simulink model "main_PETC"  (R2021a)
settings: Solver=VariableStepAuto  StartTime=0.0  StopTime=10  FixedStep=1e-4  RelTol=1e-3
InitFcn:
  | run('Parameter.m')
values from neighbouring files (symbols this model uses):
  cp = 1    [Parameter.m]
  cv = 5    [Parameter.m]
  cw = 5    [Parameter.m]
  fref = 60    [Parameter.m]
  Lc1 = 0.35e-3    (= 0.00035)    [Parameter.m]
  Lc2 = 0.35e-3    (= 0.00035)    [Parameter.m]
  Lc3 = 0.35e-3    (= 0.00035)    [Parameter.m]
  Lc4 = 0.35e-3    (= 0.00035)    [Parameter.m]
  Lt12 = 318e-6    (= 0.000318)    [Parameter.m]
  Lt23 = 1847e-6    (= 0.001847)    [Parameter.m]
  Lt34 = 318e-6    (= 0.000318)    [Parameter.m]
  Mp1 = 9.4e-5    (= 9.4e-05)    [Parameter.m]
  Mp2 = 9.4e-5    (= 9.4e-05)    [Parameter.m]
  Mp3 = 12.5e-5    (= 0.000125)    [Parameter.m]
  Mp4 = 12.5e-5    (= 0.000125)    [Parameter.m]
  Nq1 = 1.3e-3    (= 0.0013)    [Parameter.m]
  Nq2 = 1.3e-3    (= 0.0013)    [Parameter.m]
  Nq3 = 1.5e-3    (= 0.0015)    [Parameter.m]
  Nq4 = 1.5e-3    (= 0.0015)    [Parameter.m]
  Rc1 = 0.03    [Parameter.m]
  Rc2 = 0.03    [Parameter.m]
  Rc3 = 0.03    [Parameter.m]
  Rc4 = 0.03    [Parameter.m]
  Rt12 = 0.23    [Parameter.m]
  Rt23 = 0.35    [Parameter.m]
  Rt34 = 0.23    [Parameter.m]
  t2 = 1    [Parameter.m]    (also in wvpq_PETC.m)
  t3 = 10    [Parameter.m]
  t4 = 20    [Parameter.m]    (also in wvpq_PETC.m = 21)
  t5 = 35    [Parameter.m]    (also in wvpq_PETC.m = 33)
  t6 = 40    [Parameter.m]    (also in wvpq_PETC.m = 35)
  Uo = 220*sqrt(2)    [Parameter.m]
  vref = 380    [Parameter.m]
  wc = 31.4    [Parameter.m]
  wref = 2*pi*fref    (= 376.991118431)    [Parameter.m]
undefined symbols (not defined in the file or in its folder): gcbh, sps_rtmsupport
libraries: spsControlledVoltageSourceLib x12, spsAlphaBetaZerotodq0Lib x12, eeGeneralControl x8, spsThreePhaseSeriesRLCBranchLib x7, spsGroundLib x4, spsThreePhaseVIMeasurementLib x4, spsThreePhaseBreakerLib x4, spsPLL3phLib x4, spsThreePhaseSeriesRLCLoadLib x3, spspowerguiLib x1
(part 1 of 2)
settings Model: Creator=Li Ding  LastModifiedBy=服务器

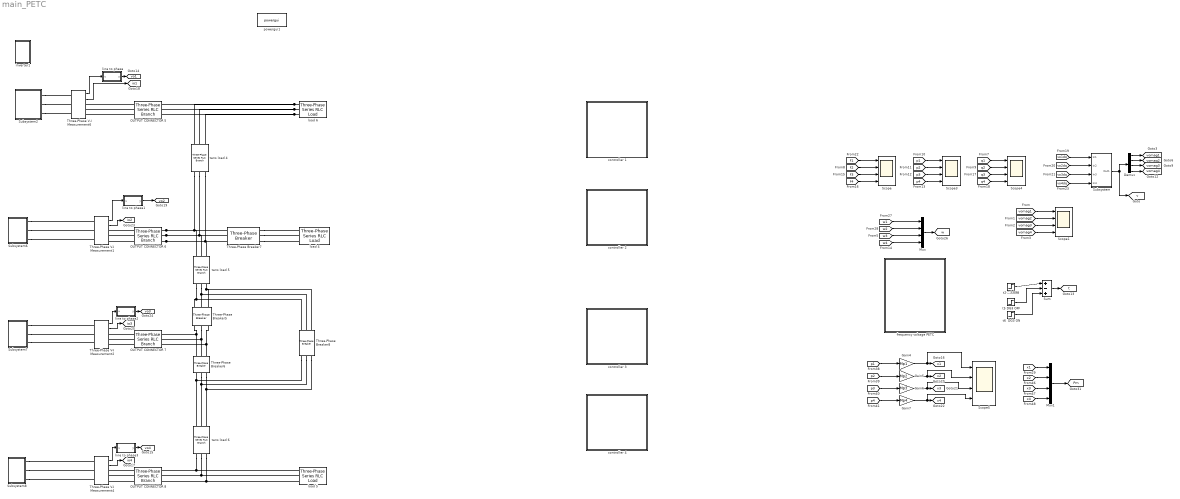
== system main_PETC ==
  Demux : Demux
  Gain4 : Gain  Gain=Mp1
  Gain5 : Gain  Gain=Mp2
  Gain6 : Gain  Gain=Mp3
  Gain7 : Gain  Gain=Mp4
  Mux : Mux
  Mux1 : Mux
  OUTPUT CONNECTOR 5 : spsThreePhaseSeriesRLCBranchLib/Three-Phase Series RLC Branch  LConnTagsString=A|B|C  RConnTagsString=A|B|C  BranchType=RL  Resistance=Rc1  Inductance=Lc1  Capacitance=1e-6  Measurements=None
  OUTPUT CONNECTOR 6 : spsThreePhaseSeriesRLCBranchLib/Three-Phase Series RLC Branch  LConnTagsString=A|B|C  RConnTagsString=A|B|C  BranchType=RL  Resistance=Rc2  Inductance=Lc2  Capacitance=1e-6  Measurements=None
  OUTPUT CONNECTOR 7 : spsThreePhaseSeriesRLCBranchLib/Three-Phase Series RLC Branch  LConnTagsString=A|B|C  RConnTagsString=A|B|C  BranchType=RL  Resistance=Rc3  Inductance=Lc3  Capacitance=1e-6  Measurements=None
  OUTPUT CONNECTOR 8 : spsThreePhaseSeriesRLCBranchLib/Three-Phase Series RLC Branch  LConnTagsString=A|B|C  RConnTagsString=A|B|C  BranchType=RL  Resistance=Rc4  Inductance=Lc4  Capacitance=1e-6  Measurements=None
  Scope{,1,3..5} (5 alike) : Scope  NumInputPorts=4
  Subsystem : Subsystem
  Subsystem2 : Subsystem
  Subsystem6 : Subsystem
  Subsystem7 : Subsystem
  Subsystem8 : Subsystem
  Sum : Sum  Inputs=|+-+
  Three-Phase V-I Measurement{1..2,4,6} (4 alike) : spsThreePhaseVIMeasurementLib/Three-Phase V-I Measurement  VoltageMeasurement=phase-to-phase  SetLabelV=off  LabelV=Vabc  Vpu=off  VpuLL=off  CurrentMeasurement=yes  SetLabelI=off  LabelI=Iabc  Ipu=off  Pbase=100e6  Vbase=500e3  OutputType=Complex  PhasorSimulation=off  PSBequivalent=0
  Three-Phase Breaker5 : spsThreePhaseBreakerLib/Three-Phase Breaker  InitialState=closed  SwitchA=on  SwitchB=on  SwitchC=on  SwitchTimes=[t5 t6]  External=off  BreakerResistance=0.01  SnubberResistance=1e6  SnubberCapacitance=inf  Measurements=None
  Three-Phase Breaker6 : spsThreePhaseBreakerLib/Three-Phase Breaker  InitialState=closed  SwitchA=on  SwitchB=on  SwitchC=on  SwitchTimes=[t5 t6]  External=off  BreakerResistance=0.01  SnubberResistance=1e6  SnubberCapacitance=inf  Measurements=None
  Three-Phase Breaker7 : spsThreePhaseBreakerLib/Three-Phase Breaker  InitialState=open  SwitchA=on  SwitchB=on  SwitchC=on  SwitchTimes=[t3 t4]  External=off  BreakerResistance=0.01  SnubberResistance=1e6  SnubberCapacitance=inf  Measurements=None
  Three-Phase Breaker8 : spsThreePhaseBreakerLib/Three-Phase Breaker  InitialState=open  SwitchA=on  SwitchB=on  SwitchC=on  SwitchTimes=[t5 t6]  External=off  BreakerResistance=0.01  SnubberResistance=1e6  SnubberCapacitance=inf  Measurements=None
  controller 1 : Subsystem
  controller 2 : Subsystem
  controller 3 : Subsystem
  controller 4 : Subsystem
  frequency voltage PETC : Subsystem
  inverter1 : Subsystem
  line to phase : MATLAB Function  TreatAsAtomicUnit=on
  line to phase1 : MATLAB Function  TreatAsAtomicUnit=on
  line to phase2 : MATLAB Function  TreatAsAtomicUnit=on
  line to phase3 : MATLAB Function  TreatAsAtomicUnit=on
  load 4 : spsThreePhaseSeriesRLCLoadLib/Three-Phase Series RLC Load  LConnTagsString=A|B|C  Configuration=Y (grounded)  NominalVoltage=vref  Vabc=[1e3 1e3 1e3]  Vabcp=[1e3 1e3 1e3]  NominalFrequency=fref  UnbalancedPower=off  ActivePower=PL2  InductivePower=QL2  CapacitivePower=0  Pabc=[10e3 9e3 11e3]  QLabc=[100 90 110]  QCabc=[100 90 110]  Pabcp=[10e3 9e3 11e3]  QLabcp=[100 90 110]  QCabcp=[100 90 110]  Measurements=None  LoadType=constant Z
  load 5 : spsThreePhaseSeriesRLCLoadLib/Three-Phase Series RLC Load  LConnTagsString=A|B|C  Configuration=Y (grounded)  NominalVoltage=vref  Vabc=[1e3 1e3 1e3]  Vabcp=[1e3 1e3 1e3]  NominalFrequency=fref  UnbalancedPower=off  ActivePower=PL4  InductivePower=QL4  CapacitivePower=0  Pabc=[10e3 9e3 11e3]  QLabc=[100 90 110]  QCabc=[100 90 110]  Pabcp=[10e3 9e3 11e3]  QLabcp=[100 90 110]  QCabcp=[100 90 110]  Measurements=None  LoadType=constant Z
  load 6 : spsThreePhaseSeriesRLCLoadLib/Three-Phase Series RLC Load  LConnTagsString=A|B|C  Configuration=Y (grounded)  NominalVoltage=vref  Vabc=[1e3 1e3 1e3]  Vabcp=[1e3 1e3 1e3]  NominalFrequency=fref  UnbalancedPower=off  ActivePower=PL1  InductivePower=QL1  CapacitivePower=0  Pabc=[10e3 9e3 11e3]  QLabc=[100 90 110]  QCabc=[100 90 110]  Pabcp=[10e3 9e3 11e3]  QLabcp=[100 90 110]  QCabcp=[100 90 110]  Measurements=None  LoadType=constant Z
  powergui1 : spspowerguiLib/powergui  Priority=1  SimulationMode=Discrete  SampleTime=50e-6  frequency=60  Iterations=50  frequencyindice=0  Pbase=100e6  ErrMax=1e-4  UnitsV=kV  UnitsW=MW  buscounter=0  FunctionMessages=off  echomessages=off  EnableUseOfTLC=off  CurrentSourceSwitches=off  DisableSnubberDevices=off  DisableRonSwitches=off  DisableVfSwitches=off  DisplayEquations=off  AutomaticDiscreteSolvers=off  SolverType=Tustin/Backward Euler (TBE)  Interpol=off  ExternalGateDelay=off  methode=off  Ts=100  x0status=blocks  SPID=on  SwTol=0  HookPort=off  NonlinearTolerance=1e-4  nMaxIteration=100  ContinueOnMaxIteration=off  RestoreLinks=warning  ResistiveCurrentMeasurement=off  Frange=[0:2:500]  Ylog=off  Xlog=on  ShowGrid=off  save=off  variable=ZData  structure=0  ZoomFFT=off  StartTime=0.0  cycles=1  DisplayStyle=1  fundamental=60  FreqAxis=off  MaxFrequency=1000  frequencyindicesteady=1  RmsSteady=1  display=off
  t2-二次控制 : Step  Time=t2  SampleTime=0
  t5 DG3 OFF : Step  Time=t5  SampleTime=0
  t6  DG3 ON : Step  Time=t6  SampleTime=0
  tans load 4 : spsThreePhaseSeriesRLCBranchLib/Three-Phase Series RLC Branch  LConnTagsString=A|B|C  RConnTagsString=A|B|C  BranchType=RL  Resistance=Rt12  Inductance=Lt12  Capacitance=1e-6  Measurements=None
  tans load 5 : spsThreePhaseSeriesRLCBranchLib/Three-Phase Series RLC Branch  LConnTagsString=A|B|C  RConnTagsString=A|B|C  BranchType=RL  Resistance=Rt23  Inductance=Lt23  Capacitance=1e-6  Measurements=None
  tans load 6 : spsThreePhaseSeriesRLCBranchLib/Three-Phase Series RLC Branch  LConnTagsString=A|B|C  RConnTagsString=A|B|C  BranchType=RL  Resistance=Rt34  Inductance=Lt34  Capacitance=1e-6  Measurements=None
  tag scope: Pm=global, io1=global, io2=global, io3=global, io4=global, t=global, v=global, vo1=global, vo2=global, vo3=global, vo4=global, vomag1=global, vomag2=global, vomag3=global, vomag4=global, w=global, x1=global, x2=global, x3=global, x4=global
  wires:
  [f3] -> Scope/3
  [f2] -> Scope/2
  [f1] -> Scope/1
  [f4] -> Scope/4
  [p4] -> Scope3/4
  [q1] -> Scope4/1
  [q4] -> Scope4/4
  [p2] -> Scope3/2
  [q2] -> Scope4/2
  [p1] -> Scope3/1
  [p3] -> Scope3/3
  [q3] -> Scope4/3
  [w1] -> Mux/1
  [w2] -> Mux/2
  [w3] -> Mux/3
  [w4] -> Mux/4
  Mux/1 -> [w]
  [p1] -> Gain4/1
  [p2] -> Gain5/1
  [p3] -> Gain6/1
  [p4] -> Gain7/1
  Gain7/1 -> Scope5/4, [x4]
  Gain6/1 -> Scope5/3, [x3]
  Gain5/1 -> Scope5/2, [x2]
  Gain4/1 -> Scope5/1, [x1]
  [x4] -> Mux1/4
  [x1] -> Mux1/1
  Mux1/1 -> [Pm]
  [x2] -> Mux1/2
  [x3] -> Mux1/3
  Demux/4 -> [vomag4]
  [vo3dq] -> Subsystem/3(In3)
  Demux/2 -> [vomag2]
  [vo1dq] -> Subsystem/1(In1)
  Subsystem/1(Out1) -> [v], Demux/1
  [vo2dq] -> Subsystem/2(In2)
  Demux/1 -> [vomag1]
  [vo4dq] -> Subsystem/4(In4)
  Demux/3 -> [vomag3]
  [vomag4] -> Scope1/4
  [vomag3] -> Scope1/3
  [vomag2] -> Scope1/2
  [vomag1] -> Scope1/1
  Sum/1 -> [t]
  t2-二次控制/1 -> Sum/1
  t5 DG3 OFF/1 -> Sum/2
  t6  DG3 ON/1 -> Sum/3
  Three-Phase V-I Measurement6/2 -> [io1]
  Three-Phase V-I Measurement4/1 -> line to phase3/1(u)
  Three-Phase V-I Measurement1/2 -> [io2]
  Three-Phase V-I Measurement6/1 -> line to phase/1(u)
  line to phase1/1(y) -> [vo2]
  Three-Phase V-I Measurement4/2 -> [io4]
  Three-Phase V-I Measurement1/1 -> line to phase1/1(u)
  line to phase/1(y) -> [vo1]
  line to phase2/1(y) -> [vo3]
  Three-Phase V-I Measurement2/1 -> line to phase2/1(u)
  line to phase3/1(y) -> [vo4]
  Three-Phase V-I Measurement2/2 -> [io3]
  connections:
  OUTPUT CONNECTOR 6/RConn2 -- tans load 4/RConn2 -- tans load 5/LConn2 -- Three-Phase Breaker7/LConn2
  OUTPUT CONNECTOR 6/RConn3 -- tans load 4/RConn3 -- tans load 5/LConn3 -- Three-Phase Breaker7/LConn3
  OUTPUT CONNECTOR 6/RConn1 -- tans load 4/RConn1 -- tans load 5/LConn1 -- Three-Phase Breaker7/LConn1
  tans load 5/RConn1 -- Three-Phase Breaker8/LConn1 -- Three-Phase Breaker5/LConn1
  load 5/LConn1 -- tans load 6/RConn1 -- OUTPUT CONNECTOR 8/RConn1
  load 5/LConn3 -- tans load 6/RConn3 -- OUTPUT CONNECTOR 8/RConn3
  load 5/LConn2 -- tans load 6/RConn2 -- OUTPUT CONNECTOR 8/RConn2
  Three-Phase Breaker5/RConn3 -- OUTPUT CONNECTOR 7/RConn3 -- Three-Phase Breaker6/LConn3
  load 6/LConn3 -- OUTPUT CONNECTOR 5/RConn3 -- tans load 4/LConn3
  load 6/LConn1 -- OUTPUT CONNECTOR 5/RConn1 -- tans load 4/LConn1
  tans load 5/RConn2 -- Three-Phase Breaker8/LConn2 -- Three-Phase Breaker5/LConn2
  tans load 5/RConn3 -- Three-Phase Breaker8/LConn3 -- Three-Phase Breaker5/LConn3
  Three-Phase Breaker6/LConn2 -- OUTPUT CONNECTOR 7/RConn2 -- Three-Phase Breaker5/RConn2
  load 6/LConn2 -- OUTPUT CONNECTOR 5/RConn2 -- tans load 4/LConn2
  Three-Phase Breaker5/RConn1 -- OUTPUT CONNECTOR 7/RConn1 -- Three-Phase Breaker6/LConn1
  Subsystem2/LConn2 -- Three-Phase V-I Measurement6/LConn2
  OUTPUT CONNECTOR 8/LConn1 -- Three-Phase V-I Measurement4/RConn1
  Subsystem2/LConn1 -- Three-Phase V-I Measurement6/LConn1
  Three-Phase Breaker6/RConn3 -- Three-Phase Breaker8/RConn3 -- tans load 6/LConn3
  Subsystem8/LConn1 -- Three-Phase V-I Measurement4/LConn1
  OUTPUT CONNECTOR 8/LConn3 -- Three-Phase V-I Measurement4/RConn3
  OUTPUT CONNECTOR 6/LConn3 -- Three-Phase V-I Measurement1/RConn3
  Subsystem7/LConn1 -- Three-Phase V-I Measurement2/LConn1
  Three-Phase Breaker7/RConn2 -- load 4/LConn2
  Subsystem6/LConn1 -- Three-Phase V-I Measurement1/LConn1
  Subsystem7/LConn3 -- Three-Phase V-I Measurement2/LConn3
  Subsystem6/LConn2 -- Three-Phase V-I Measurement1/LConn2
  Three-Phase Breaker7/RConn1 -- load 4/LConn1
  OUTPUT CONNECTOR 7/LConn3 -- Three-Phase V-I Measurement2/RConn3
  OUTPUT CONNECTOR 7/LConn1 -- Three-Phase V-I Measurement2/RConn1
  Three-Phase Breaker7/RConn3 -- load 4/LConn3
  Subsystem6/LConn3 -- Three-Phase V-I Measurement1/LConn3
  Three-Phase Breaker6/RConn2 -- Three-Phase Breaker8/RConn2 -- tans load 6/LConn2
  Subsystem8/LConn3 -- Three-Phase V-I Measurement4/LConn3
  OUTPUT CONNECTOR 5/LConn2 -- Three-Phase V-I Measurement6/RConn2
  OUTPUT CONNECTOR 8/LConn2 -- Three-Phase V-I Measurement4/RConn2
  OUTPUT CONNECTOR 7/LConn2 -- Three-Phase V-I Measurement2/RConn2
  Subsystem7/LConn2 -- Three-Phase V-I Measurement2/LConn2
  Subsystem2/LConn3 -- Three-Phase V-I Measurement6/LConn3
  OUTPUT CONNECTOR 6/LConn1 -- Three-Phase V-I Measurement1/RConn1
  OUTPUT CONNECTOR 5/LConn3 -- Three-Phase V-I Measurement6/RConn3
  OUTPUT CONNECTOR 5/LConn1 -- Three-Phase V-I Measurement6/RConn1
  Subsystem8/LConn2 -- Three-Phase V-I Measurement4/LConn2
  OUTPUT CONNECTOR 6/LConn2 -- Three-Phase V-I Measurement1/RConn2
  tans load 6/LConn1 -- Three-Phase Breaker8/RConn1 -- Three-Phase Breaker6/RConn1

== system main_PETC/Subsystem ==
  In1 : Inport
  In2 : Inport  Port=2
  In3 : Inport  Port=3
  In4 : Inport  Port=4
  Mux : Mux
  Scope : Scope
  Selector{,1..3} (4 alike) : Selector  InputPortWidth=2  IndexOptions=Index vector (dialog)  Indices=[1]  OutputSizes=1
  Transfer Fcn{,2,4,6} (4 alike) : TransferFcn  Numerator=[200]  Denominator=[1 200]
  Out1 : Outport
  wires:
  Selector1/1 -> Transfer Fcn2/1
  Selector3/1 -> Transfer Fcn6/1
  In4/1 -> Selector3/1
  Selector2/1 -> Transfer Fcn4/1
  Mux/1 -> Out1/1
  In3/1 -> Selector2/1
  In2/1 -> Selector1/1
  In1/1 -> Selector/1
  Transfer Fcn/1 -> Mux/1
  Transfer Fcn2/1 -> Mux/2
  Transfer Fcn4/1 -> Mux/3
  Transfer Fcn6/1 -> Mux/4
  Selector/1 -> Scope/1, Transfer Fcn/1

== system main_PETC/Subsystem2 ==
  Controlled Voltage Source : spsControlledVoltageSourceLib/Controlled Voltage Source  Initialize=on  Source_Type=AC  Amplitude=Uo  Phase=0  Frequency=fref  Measurements=None
  Controlled Voltage Source1 : spsControlledVoltageSourceLib/Controlled Voltage Source  Initialize=on  Source_Type=AC  Amplitude=Uo  Phase=120  Frequency=fref  Measurements=None
  Controlled Voltage Source2 : spsControlledVoltageSourceLib/Controlled Voltage Source  Initialize=on  Source_Type=AC  Amplitude=Uo  Phase=240  Frequency=fref  Measurements=None
  Demux : Demux  Outputs=3
  Ground : spsGroundLib/Ground  LConnTagsString=a
  +1 : PMIOPort  Side=Left
  +2 : PMIOPort  Port=2  Side=Left
  +3 : PMIOPort  Port=3  Side=Left
  wires:
  Demux/1 -> Controlled Voltage Source/1
  Demux/2 -> Controlled Voltage Source1/1
  Demux/3 -> Controlled Voltage Source2/1
  [VOL1] -> Demux/1
  connections:
  Controlled Voltage Source/RConn1 -- +1/RConn1
  Controlled Voltage Source1/RConn1 -- +2/RConn1
  Controlled Voltage Source2/RConn1 -- +3/RConn1
  Controlled Voltage Source2/LConn1 -- Ground/LConn1 -- Controlled Voltage Source/LConn1 -- Controlled Voltage Source1/LConn1

== system main_PETC/Subsystem6 ==
  Controlled Voltage Source : spsControlledVoltageSourceLib/Controlled Voltage Source  Initialize=on  Source_Type=AC  Amplitude=Uo  Phase=0  Frequency=fref  Measurements=None
  Controlled Voltage Source1 : spsControlledVoltageSourceLib/Controlled Voltage Source  Initialize=on  Source_Type=AC  Amplitude=Uo  Phase=120  Frequency=fref  Measurements=None
  Controlled Voltage Source2 : spsControlledVoltageSourceLib/Controlled Voltage Source  Initialize=on  Source_Type=AC  Amplitude=Uo  Phase=240  Frequency=fref  Measurements=None
  Demux : Demux  Outputs=3
  Ground : spsGroundLib/Ground  LConnTagsString=a
  +1 : PMIOPort  Side=Left
  +2 : PMIOPort  Port=2  Side=Left
  +3 : PMIOPort  Port=3  Side=Left
  wires:
  Demux/1 -> Controlled Voltage Source/1
  Demux/2 -> Controlled Voltage Source1/1
  Demux/3 -> Controlled Voltage Source2/1
  [VOL2] -> Demux/1
  connections:
  Controlled Voltage Source/RConn1 -- +1/RConn1
  Controlled Voltage Source1/RConn1 -- +2/RConn1
  Controlled Voltage Source2/RConn1 -- +3/RConn1
  Controlled Voltage Source/LConn1 -- Controlled Voltage Source1/LConn1 -- Controlled Voltage Source2/LConn1 -- Ground/LConn1

== system main_PETC/Subsystem7 ==
  Controlled Voltage Source : spsControlledVoltageSourceLib/Controlled Voltage Source  Initialize=on  Source_Type=AC  Amplitude=Uo  Phase=0  Frequency=fref  Measurements=None
  Controlled Voltage Source1 : spsControlledVoltageSourceLib/Controlled Voltage Source  Initialize=on  Source_Type=AC  Amplitude=Uo  Phase=120  Frequency=fref  Measurements=None
  Controlled Voltage Source2 : spsControlledVoltageSourceLib/Controlled Voltage Source  Initialize=on  Source_Type=AC  Amplitude=Uo  Phase=240  Frequency=fref  Measurements=None
  Demux : Demux  Outputs=3
  Ground : spsGroundLib/Ground  LConnTagsString=a
  +1 : PMIOPort  Side=Left
  +2 : PMIOPort  Port=2  Side=Left
  +3 : PMIOPort  Port=3  Side=Left
  wires:
  Demux/1 -> Controlled Voltage Source/1
  Demux/2 -> Controlled Voltage Source1/1
  Demux/3 -> Controlled Voltage Source2/1
  [VOL3] -> Demux/1
  connections:
  Controlled Voltage Source/RConn1 -- +1/RConn1
  Controlled Voltage Source1/RConn1 -- +2/RConn1
  Controlled Voltage Source2/RConn1 -- +3/RConn1
  Controlled Voltage Source/LConn1 -- Controlled Voltage Source1/LConn1 -- Controlled Voltage Source2/LConn1 -- Ground/LConn1

== system main_PETC/Subsystem8 ==
  Controlled Voltage Source : spsControlledVoltageSourceLib/Controlled Voltage Source  Initialize=on  Source_Type=AC  Amplitude=Uo  Phase=0  Frequency=fref  Measurements=None
  Controlled Voltage Source1 : spsControlledVoltageSourceLib/Controlled Voltage Source  Initialize=on  Source_Type=AC  Amplitude=Uo  Phase=120  Frequency=fref  Measurements=None
  Controlled Voltage Source2 : spsControlledVoltageSourceLib/Controlled Voltage Source  Initialize=on  Source_Type=AC  Amplitude=Uo  Phase=240  Frequency=fref  Measurements=None
  Demux : Demux  Outputs=3
  Ground : spsGroundLib/Ground  LConnTagsString=a
  +1 : PMIOPort  Side=Left
  +2 : PMIOPort  Port=2  Side=Left
  +3 : PMIOPort  Port=3  Side=Left
  wires:
  Demux/1 -> Controlled Voltage Source/1
  Demux/2 -> Controlled Voltage Source1/1
  Demux/3 -> Controlled Voltage Source2/1
  [VOL4] -> Demux/1
  connections:
  Controlled Voltage Source/RConn1 -- +1/RConn1
  Controlled Voltage Source1/RConn1 -- +2/RConn1
  Controlled Voltage Source2/RConn1 -- +3/RConn1
  Controlled Voltage Source/LConn1 -- Controlled Voltage Source1/LConn1 -- Controlled Voltage Source2/LConn1 -- Ground/LConn1

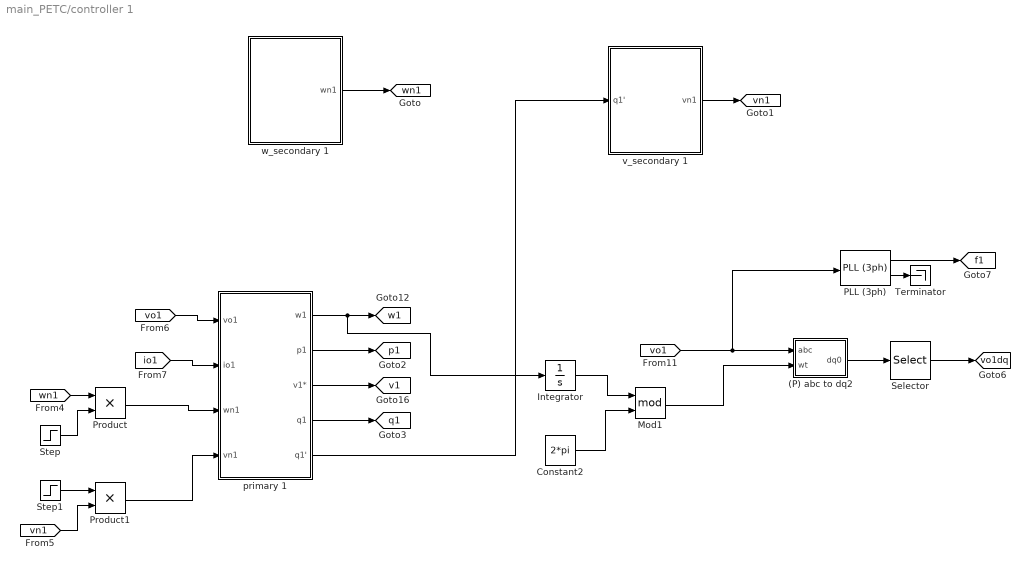
== system main_PETC/controller 1 ==
  (P) abc to dq2 : Subsystem  AncestorBlock=powerlib_meascontrol/Transformations/abc to dq0  DialogController=POWERSYS.PowerSysDialog  LoadFcn=sps_rtmsupport('LoadFcn', gcbh);  StartFcn=sps_rtmsupport('StartFcn', gcbh);  StopFcn=sps_rtmsupport('StopFcn', gcbh);  mask(abc to dq0 Transformation){Alignment=90 degrees behind phase A axis}
      mask prompts: Alignment "Rotating frame alignment at wt=0:"
      mask help:
      | Perform a Park transformation from a three-phase (abc) signal to a dq0 rotating reference frame. Angular position of the rotating frame is given by input wt (rad).
      |
      | When the rotating frame alignment at wt=0 is 90 degrees behind phase A axis, a positive-sequence signal with Mag=1 & Phase=0 degrees yields the following dq values: d=1, q=0.
      mask init:
      | str=cat(2,gcb,'/Alpha-Beta-Zero to dq0');
      | if Alignment==1
      |     set_param(str,'Alignment','Aligned with phase A axis');
      | else
      |     set_param(str,'Alignment','90 degrees behind phase A axis');
      | end
      settings: CopyFcn=sps_rtmsupport('CopyFcn', gcbh);  DeleteFcn=sps_rtmsupport('DeleteFcn', gcbh);  UndoDeleteFcn=sps_rtmsupport('UndoDeleteFcn', gcbh);  ModelCloseFcn=sps_rtmsupport('ModelCloseFcn', gcbh);  PreSaveFcn=sps_rtmsupport('PreSaveFcn', gcbh);  PostSaveFcn=sps_rtmsupport('PostSaveFcn', gcbh);  NameChangeFcn=sps_rtmsupport('NameChangeFcn', gcbh);  PreCopyFcn=sps_rtmsupport('PreCopyFcn', gcbh);  OpenFcn=sps_rtmsupport('OpenFcn', gcbh, [1]);  CloseFcn=sps_rtmsupport('CloseFcn', gcbh);  PreDeleteFcn=sps_rtmsupport('PreDeleteFcn', gcbh);
      mask Help: helpview(psbhelp);
      mask TypeOptions Alignment: Aligned with phase A axis | 90 degrees behind phase A axis
      mask Display:
      | plot([0 1], [0,1])
      | port_label('input', 1, 'abc')
      | port_label('input', 2, 'wt')
      | port_label('output', 1, 'dq0')
  Constant2 : Constant  Value=2*pi
  Integrator : Integrator
  Mod1 : Math  Operator=mod  SaturateOnIntegerOverflow=on
  PLL (3ph) : spsPLL3phLib/PLL (3ph)  Fmin=45  Par_Init=[0, fref]  ParK=[180, 3200, 1]  TcD=1e-4  MaxRateChangeFreq=12  FilterCutOffFreq=25  Ts=0  AGC=on
  Product : Product
  Product1 : Product
  Selector : Selector  InputPortWidth=3  IndexOptions=Index vector (dialog)  Indices=[1 2]  OutputSizes=1
  Step : Step  Time=t2  SampleTime=0
  Step1 : Step  Time=t2  SampleTime=0
  Terminator : Terminator
  primary 1 : Subsystem
  v_secondary 1 : Subsystem
  w_secondary 1 : Subsystem
  tag scope: f1=global, p1=global, q1=global, v1=global, vn1=global, vo1dq=global, w1=global, wn1=global
  wires:
  w_secondary 1/1(wn1) -> [wn1]
  v_secondary 1/1(vn1) -> [vn1]
  primary 1/5(q1') -> v_secondary 1/1(q1')
  PLL (3ph)/2 -> Terminator/1
  Product/1 -> primary 1/3(wn1)
  (P) abc to dq2/1(dq0) -> Selector/1
  primary 1/3(v1*) -> [v1]
  Mod1/1 -> (P) abc to dq2/2(wt)
  Step/1 -> Product/2
  primary 1/4(q1) -> [q1]
  [vn1] -> Product1/2
  Product1/1 -> primary 1/4(vn1)
  primary 1/1(w1) -> Integrator/1, [w1]
  [vo1] -> (P) abc to dq2/1(abc), PLL (3ph)/1
  Constant2/1 -> Mod1/2
  Step1/1 -> Product1/1
  Integrator/1 -> Mod1/1
  [vo1] -> primary 1/1(vo1)
  primary 1/2(p1) -> [p1]
  PLL (3ph)/1 -> [f1]
  Selector/1 -> [vo1dq]
  [wn1] -> Product/1
  [io1] -> primary 1/2(io1)

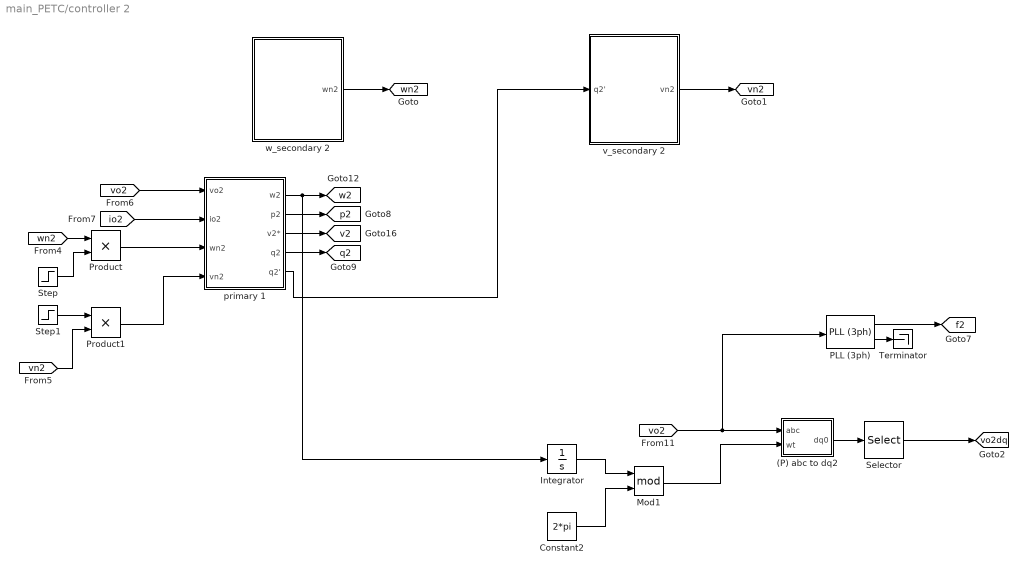
== system main_PETC/controller 2 ==
  (P) abc to dq2 : Subsystem  AncestorBlock=powerlib_meascontrol/Transformations/abc to dq0  DialogController=POWERSYS.PowerSysDialog  LoadFcn=sps_rtmsupport('LoadFcn', gcbh);  StartFcn=sps_rtmsupport('StartFcn', gcbh);  StopFcn=sps_rtmsupport('StopFcn', gcbh);  mask(abc to dq0 Transformation){Alignment=90 degrees behind phase A axis}
      mask prompts: Alignment "Rotating frame alignment at wt=0:"
      mask help:
      | Perform a Park transformation from a three-phase (abc) signal to a dq0 rotating reference frame. Angular position of the rotating frame is given by input wt (rad).
      |
      | When the rotating frame alignment at wt=0 is 90 degrees behind phase A axis, a positive-sequence signal with Mag=1 & Phase=0 degrees yields the following dq values: d=1, q=0.
      mask init:
      | str=cat(2,gcb,'/Alpha-Beta-Zero to dq0');
      | if Alignment==1
      |     set_param(str,'Alignment','Aligned with phase A axis');
      | else
      |     set_param(str,'Alignment','90 degrees behind phase A axis');
      | end
      settings: CopyFcn=sps_rtmsupport('CopyFcn', gcbh);  DeleteFcn=sps_rtmsupport('DeleteFcn', gcbh);  UndoDeleteFcn=sps_rtmsupport('UndoDeleteFcn', gcbh);  ModelCloseFcn=sps_rtmsupport('ModelCloseFcn', gcbh);  PreSaveFcn=sps_rtmsupport('PreSaveFcn', gcbh);  PostSaveFcn=sps_rtmsupport('PostSaveFcn', gcbh);  NameChangeFcn=sps_rtmsupport('NameChangeFcn', gcbh);  PreCopyFcn=sps_rtmsupport('PreCopyFcn', gcbh);  OpenFcn=sps_rtmsupport('OpenFcn', gcbh, [1]);  CloseFcn=sps_rtmsupport('CloseFcn', gcbh);  PreDeleteFcn=sps_rtmsupport('PreDeleteFcn', gcbh);
      mask Help: helpview(psbhelp);
      mask TypeOptions Alignment: Aligned with phase A axis | 90 degrees behind phase A axis
      mask Display:
      | plot([0 1], [0,1])
      | port_label('input', 1, 'abc')
      | port_label('input', 2, 'wt')
      | port_label('output', 1, 'dq0')
  Constant2 : Constant  Value=2*pi
  Integrator : Integrator
  Mod1 : Math  Operator=mod  SaturateOnIntegerOverflow=on
  PLL (3ph) : spsPLL3phLib/PLL (3ph)  Fmin=45  Par_Init=[0, 60]  ParK=[180, 3200, 1]  TcD=1e-4  MaxRateChangeFreq=12  FilterCutOffFreq=25  Ts=0  AGC=on
  Product : Product
  Product1 : Product
  Selector : Selector  InputPortWidth=3  IndexOptions=Index vector (dialog)  Indices=[1 2]  OutputSizes=1
  Step : Step  Time=t2  SampleTime=0
  Step1 : Step  Time=t2  SampleTime=0
  Terminator : Terminator
  primary 1 : Subsystem
  v_secondary 2 : Subsystem
  w_secondary 2 : Subsystem
  tag scope: f2=global, p2=global, q2=global, v2=global, vn2=global, vo2dq=global, w2=global, wn2=global
  wires:
  w_secondary 2/1(wn2) -> [wn2]
  v_secondary 2/1(vn2) -> [vn2]
  PLL (3ph)/2 -> Terminator/1
  primary 1/3(v2*) -> [v2]
  Step1/1 -> Product1/1
  Step/1 -> Product/2
  primary 1/2(p2) -> [p2]
  Product1/1 -> primary 1/4(vn2)
  [vn2] -> Product1/2
  primary 1/4(q2) -> [q2]
  [vo2] -> primary 1/1(vo2)
  PLL (3ph)/1 -> [f2]
  [io2] -> primary 1/2(io2)
  Product/1 -> primary 1/3(wn2)
  primary 1/5(q2') -> v_secondary 2/1(q2')
  Integrator/1 -> Mod1/1
  [wn2] -> Product/1
  (P) abc to dq2/1(dq0) -> Selector/1
  Constant2/1 -> Mod1/2
  Mod1/1 -> (P) abc to dq2/2(wt)
  [vo2] -> (P) abc to dq2/1(abc), PLL (3ph)/1
  primary 1/1(w2) -> [w2], Integrator/1
  Selector/1 -> [vo2dq]

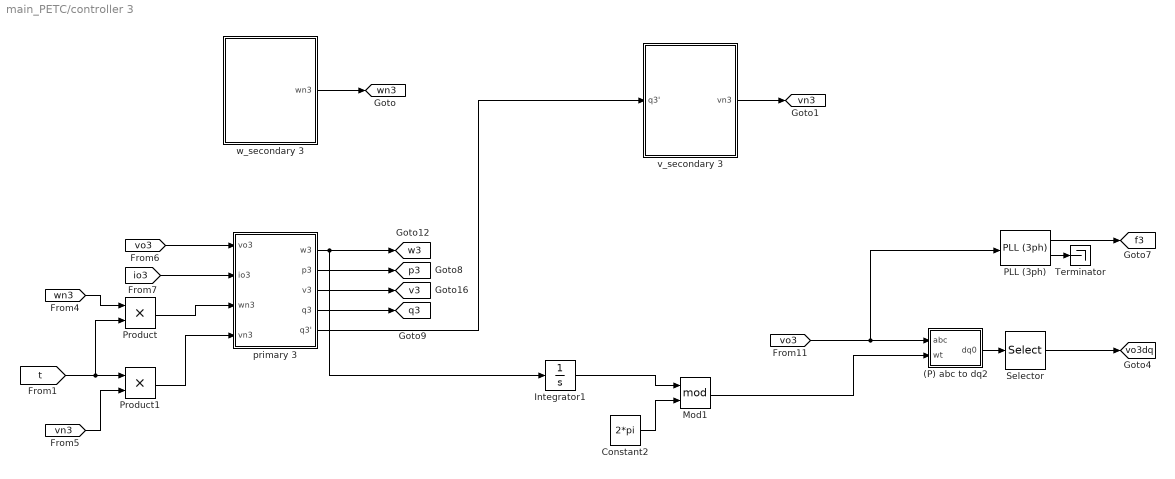
== system main_PETC/controller 3 ==
  (P) abc to dq2 : Subsystem  AncestorBlock=powerlib_meascontrol/Transformations/abc to dq0  DialogController=POWERSYS.PowerSysDialog  LoadFcn=sps_rtmsupport('LoadFcn', gcbh);  StartFcn=sps_rtmsupport('StartFcn', gcbh);  StopFcn=sps_rtmsupport('StopFcn', gcbh);  mask(abc to dq0 Transformation){Alignment=90 degrees behind phase A axis}
      mask prompts: Alignment "Rotating frame alignment at wt=0:"
      mask help:
      | Perform a Park transformation from a three-phase (abc) signal to a dq0 rotating reference frame. Angular position of the rotating frame is given by input wt (rad).
      |
      | When the rotating frame alignment at wt=0 is 90 degrees behind phase A axis, a positive-sequence signal with Mag=1 & Phase=0 degrees yields the following dq values: d=1, q=0.
      mask init:
      | str=cat(2,gcb,'/Alpha-Beta-Zero to dq0');
      | if Alignment==1
      |     set_param(str,'Alignment','Aligned with phase A axis');
      | else
      |     set_param(str,'Alignment','90 degrees behind phase A axis');
      | end
      settings: CopyFcn=sps_rtmsupport('CopyFcn', gcbh);  DeleteFcn=sps_rtmsupport('DeleteFcn', gcbh);  UndoDeleteFcn=sps_rtmsupport('UndoDeleteFcn', gcbh);  ModelCloseFcn=sps_rtmsupport('ModelCloseFcn', gcbh);  PreSaveFcn=sps_rtmsupport('PreSaveFcn', gcbh);  PostSaveFcn=sps_rtmsupport('PostSaveFcn', gcbh);  NameChangeFcn=sps_rtmsupport('NameChangeFcn', gcbh);  PreCopyFcn=sps_rtmsupport('PreCopyFcn', gcbh);  OpenFcn=sps_rtmsupport('OpenFcn', gcbh, [1]);  CloseFcn=sps_rtmsupport('CloseFcn', gcbh);  PreDeleteFcn=sps_rtmsupport('PreDeleteFcn', gcbh);
      mask Help: helpview(psbhelp);
      mask TypeOptions Alignment: Aligned with phase A axis | 90 degrees behind phase A axis
      mask Display:
      | plot([0 1], [0,1])
      | port_label('input', 1, 'abc')
      | port_label('input', 2, 'wt')
      | port_label('output', 1, 'dq0')
  Constant2 : Constant  Value=2*pi
  Integrator1 : Integrator
  Mod1 : Math  Operator=mod  SaturateOnIntegerOverflow=on
  PLL (3ph) : spsPLL3phLib/PLL (3ph)  Fmin=45  Par_Init=[0, 60]  ParK=[180, 3200, 1]  TcD=1e-4  MaxRateChangeFreq=12  FilterCutOffFreq=25  Ts=0  AGC=on
  Product : Product
  Product1 : Product
  Selector : Selector  InputPortWidth=3  IndexOptions=Index vector (dialog)  Indices=[1 2]  OutputSizes=1
  Terminator : Terminator
  primary 3 : Subsystem
  v_secondary 3 : Subsystem
  w_secondary 3 : Subsystem
  tag scope: f3=global, p3=global, q3=global, v3=global, vn3=global, vo3dq=global, w3=global, wn3=global
  wires:
  w_secondary 3/1(wn3) -> [wn3]
  v_secondary 3/1(vn3) -> [vn3]
  Integrator1/1 -> Mod1/1
  primary 3/5(q3') -> v_secondary 3/1(q3')
  [vo3] -> (P) abc to dq2/1(abc), PLL (3ph)/1
  [t] -> Product/2, Product1/1
  Mod1/1 -> (P) abc to dq2/2(wt)
  Constant2/1 -> Mod1/2
  primary 3/4(q3) -> [q3]
  Selector/1 -> [vo3dq]
  primary 3/3(v3) -> [v3]
  (P) abc to dq2/1(dq0) -> Selector/1
  PLL (3ph)/1 -> [f3]
  [vo3] -> primary 3/1(vo3)
  PLL (3ph)/2 -> Terminator/1
  primary 3/2(p3) -> [p3]
  Product/1 -> primary 3/3(wn3)
  primary 3/1(w3) -> [w3], Integrator1/1
  Product1/1 -> primary 3/4(vn3)
  [wn3] -> Product/1
  [vn3] -> Product1/2
  [io3] -> primary 3/2(io3)

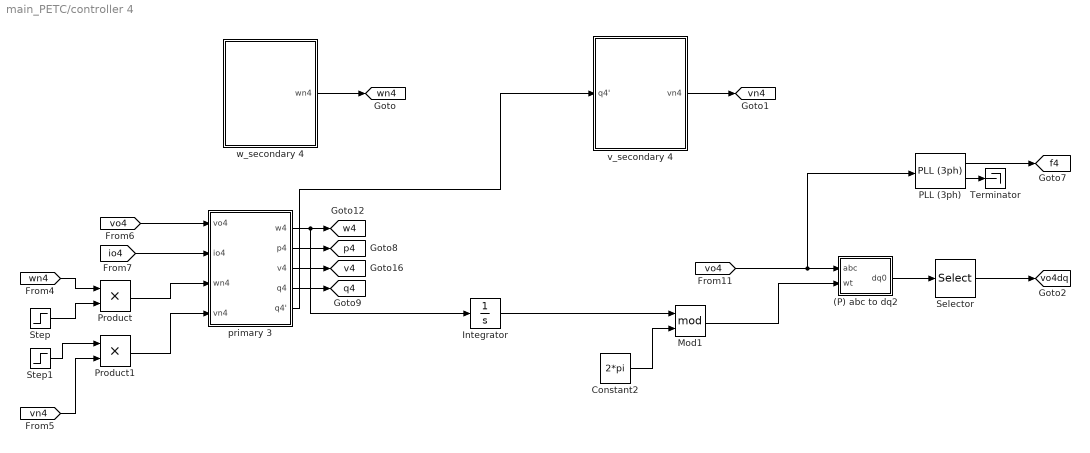
== system main_PETC/controller 4 ==
  (P) abc to dq2 : Subsystem  AncestorBlock=powerlib_meascontrol/Transformations/abc to dq0  DialogController=POWERSYS.PowerSysDialog  LoadFcn=sps_rtmsupport('LoadFcn', gcbh);  StartFcn=sps_rtmsupport('StartFcn', gcbh);  StopFcn=sps_rtmsupport('StopFcn', gcbh);  mask(abc to dq0 Transformation){Alignment=90 degrees behind phase A axis}
      mask prompts: Alignment "Rotating frame alignment at wt=0:"
      mask help:
      | Perform a Park transformation from a three-phase (abc) signal to a dq0 rotating reference frame. Angular position of the rotating frame is given by input wt (rad).
      |
      | When the rotating frame alignment at wt=0 is 90 degrees behind phase A axis, a positive-sequence signal with Mag=1 & Phase=0 degrees yields the following dq values: d=1, q=0.
      mask init:
      | str=cat(2,gcb,'/Alpha-Beta-Zero to dq0');
      | if Alignment==1
      |     set_param(str,'Alignment','Aligned with phase A axis');
      | else
      |     set_param(str,'Alignment','90 degrees behind phase A axis');
      | end
      settings: CopyFcn=sps_rtmsupport('CopyFcn', gcbh);  DeleteFcn=sps_rtmsupport('DeleteFcn', gcbh);  UndoDeleteFcn=sps_rtmsupport('UndoDeleteFcn', gcbh);  ModelCloseFcn=sps_rtmsupport('ModelCloseFcn', gcbh);  PreSaveFcn=sps_rtmsupport('PreSaveFcn', gcbh);  PostSaveFcn=sps_rtmsupport('PostSaveFcn', gcbh);  NameChangeFcn=sps_rtmsupport('NameChangeFcn', gcbh);  PreCopyFcn=sps_rtmsupport('PreCopyFcn', gcbh);  OpenFcn=sps_rtmsupport('OpenFcn', gcbh, [1]);  CloseFcn=sps_rtmsupport('CloseFcn', gcbh);  PreDeleteFcn=sps_rtmsupport('PreDeleteFcn', gcbh);
      mask Help: helpview(psbhelp);
      mask TypeOptions Alignment: Aligned with phase A axis | 90 degrees behind phase A axis
      mask Display:
      | plot([0 1], [0,1])
      | port_label('input', 1, 'abc')
      | port_label('input', 2, 'wt')
      | port_label('output', 1, 'dq0')
  Constant2 : Constant  Value=2*pi
  Integrator : Integrator
  Mod1 : Math  Operator=mod  SaturateOnIntegerOverflow=on
  PLL (3ph) : spsPLL3phLib/PLL (3ph)  Fmin=45  Par_Init=[0, 60]  ParK=[180, 3200, 1]  TcD=1e-4  MaxRateChangeFreq=12  FilterCutOffFreq=25  Ts=0  AGC=on
  Product : Product
  Product1 : Product
  Selector : Selector  InputPortWidth=3  IndexOptions=Index vector (dialog)  Indices=[1 2]  OutputSizes=1
  Step : Step  Time=t2  SampleTime=0
  Step1 : Step  Time=t2  SampleTime=0
  Terminator : Terminator
  primary 3 : Subsystem
  v_secondary 4 : Subsystem
  w_secondary 4 : Subsystem
  tag scope: f4=global, p4=global, q4=global, v4=global, vn4=global, vo4dq=global, w4=global, wn4=global
  wires:
  w_secondary 4/1(wn4) -> [wn4]
  v_secondary 4/1(vn4) -> [vn4]
  [vn4] -> Product1/2
  primary 3/2(p4) -> [p4]
  primary 3/4(q4) -> [q4]
  Product1/1 -> primary 3/4(vn4)
  Integrator/1 -> Mod1/1
  primary 3/5(q4') -> v_secondary 4/1(q4')
  [vo4] -> (P) abc to dq2/1(abc), PLL (3ph)/1
  (P) abc to dq2/1(dq0) -> Selector/1
  PLL (3ph)/1 -> [f4]
  [io4] -> primary 3/2(io4)
  Product/1 -> primary 3/3(wn4)
  PLL (3ph)/2 -> Terminator/1
  [vo4] -> primary 3/1(vo4)
  primary 3/1(w4) -> [w4], Integrator/1
  Selector/1 -> [vo4dq]
  Step/1 -> Product/2
  Mod1/1 -> (P) abc to dq2/2(wt)
  primary 3/3(v4) -> [v4]
  [wn4] -> Product/1
  Constant2/1 -> Mod1/2
  Step1/1 -> Product1/1

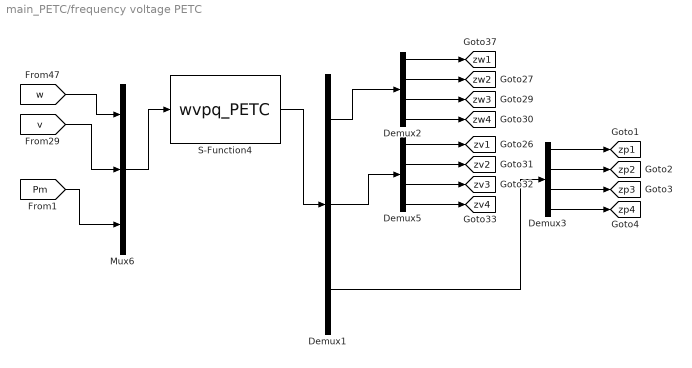
== system main_PETC/frequency voltage PETC ==
  Demux1 : Demux  Outputs=3
  Demux2 : Demux
  Demux3 : Demux
  Demux5 : Demux
  Mux6 : Mux  Inputs=3
  S-Function4 : S-Function  FunctionName=wvpq_PETC  SFunctionDeploymentMode=off  EnableBusSupport=off
  tag scope: zp1=global, zp2=global, zp3=global, zp4=global, zv1=global, zv2=global, zv3=global, zv4=global, zw1=global, zw2=global, zw3=global, zw4=global
  wires:
  Demux5/3 -> [zv3]
  [v] -> Mux6/2
  Demux2/4 -> [zw4]
  Demux2/3 -> [zw3]
  Mux6/1 -> S-Function4/1
  Demux5/1 -> [zv1]
  Demux5/4 -> [zv4]
  Demux5/2 -> [zv2]
  S-Function4/1 -> Demux1/1
  Demux1/2 -> Demux5/1
  [w] -> Mux6/1
  Demux1/1 -> Demux2/1
  Demux2/1 -> [zw1]
  Demux2/2 -> [zw2]
  [Pm] -> Mux6/3
  Demux3/3 -> [zp3]
  Demux1/3 -> Demux3/1
  Demux3/4 -> [zp4]
  Demux3/2 -> [zp2]
  Demux3/1 -> [zp1]

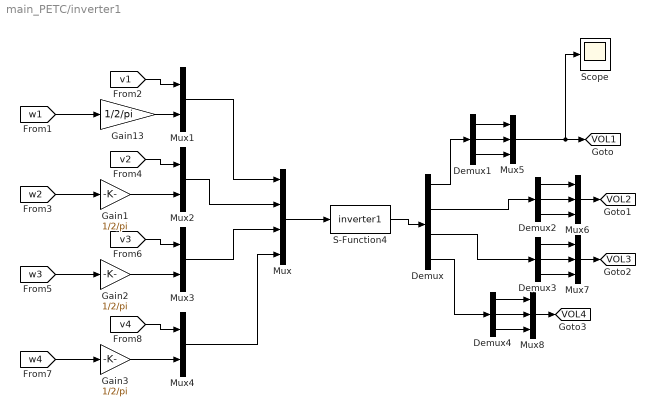
== system main_PETC/inverter1 ==
  Demux : Demux
  Demux{1..4} (4 alike) : Demux  Outputs=3
  Gain{1..3,13} (4 alike) : Gain  Gain=1/2/pi
  Mux : Mux
  Mux{1..4} (4 alike) : Mux  Inputs=2
  Mux{5..8} (4 alike) : Mux  Inputs=3
  S-Function4 : S-Function  FunctionName=inverter1  SFunctionDeploymentMode=off  EnableBusSupport=off
  Scope : Scope
  tag scope: VOL1=global, VOL2=global, VOL3=global, VOL4=global
  wires:
  Gain13/1 -> Mux1/2
  [v1] -> Mux1/1
  [w1] -> Gain13/1
  [w2] -> Gain1/1
  [v2] -> Mux2/1
  Gain1/1 -> Mux2/2
  [w3] -> Gain2/1
  [v3] -> Mux3/1
  Gain2/1 -> Mux3/2
  [w4] -> Gain3/1
  [v4] -> Mux4/1
  Gain3/1 -> Mux4/2
  Mux1/1 -> Mux/1
  Mux2/1 -> Mux/2
  Mux3/1 -> Mux/3
  Mux4/1 -> Mux/4
  Mux/1 -> S-Function4/1
  S-Function4/1 -> Demux/1
  Demux/1 -> Demux1/1
  Demux1/1 -> Mux5/1
  Demux1/2 -> Mux5/2
  Demux1/3 -> Mux5/3
  Mux5/1 -> Scope/1, [VOL1]
  Demux/2 -> Demux2/1
  Demux2/3 -> Mux6/3
  Demux2/2 -> Mux6/2
  Demux2/1 -> Mux6/1
  Mux6/1 -> [VOL2]
  Mux7/1 -> [VOL3]
  Demux3/2 -> Mux7/2
  Demux3/3 -> Mux7/3
  Demux/3 -> Demux3/1
  Demux3/1 -> Mux7/1
  Mux8/1 -> [VOL4]
  Demux4/2 -> Mux8/2
  Demux4/3 -> Mux8/3
  Demux/4 -> Demux4/1
  Demux4/1 -> Mux8/1

== system main_PETC/controller 1/(P) abc to dq2 ==
  abc : Inport  PortDimensions=3
  wt : Inport  Port=2  PortDimensions=1
  Alpha-Beta-Zero to dq0 : spsAlphaBetaZerotodq0Lib/Alpha-Beta-Zero to dq0  Alignment=90 degrees behind phase A axis
      settings: SourceProductBaseCode=PS
  abc to Alpha-Beta-Zero : Subsystem  AncestorBlock=powerlib_meascontrol/Transformations/abc to Alpha-Beta-Zero  DialogController=POWERSYS.PowerSysDialog  LoadFcn=sps_rtmsupport('LoadFcn', gcbh);  StartFcn=sps_rtmsupport('StartFcn', gcbh);  StopFcn=sps_rtmsupport('StopFcn', gcbh);  mask(abc to Alpha-Beta-Zero Transformation){}
      mask help: Perform a Clarke transformation from a three-phase (abc) signal to a alpha-beta-zero stationary reference frame.
      settings: CopyFcn=sps_rtmsupport('CopyFcn', gcbh);  DeleteFcn=sps_rtmsupport('DeleteFcn', gcbh);  UndoDeleteFcn=sps_rtmsupport('UndoDeleteFcn', gcbh);  ModelCloseFcn=sps_rtmsupport('ModelCloseFcn', gcbh);  PreSaveFcn=sps_rtmsupport('PreSaveFcn', gcbh);  PostSaveFcn=sps_rtmsupport('PostSaveFcn', gcbh);  NameChangeFcn=sps_rtmsupport('NameChangeFcn', gcbh);  PreCopyFcn=sps_rtmsupport('PreCopyFcn', gcbh);  OpenFcn=sps_rtmsupport('OpenFcn', gcbh, []);  CloseFcn=sps_rtmsupport('CloseFcn', gcbh);  PreDeleteFcn=sps_rtmsupport('PreDeleteFcn', gcbh);
      mask Help: helpview(psbhelp);
      mask Display:
      | plot([0 1], [0,1])
      | text(0.15,0.7,'abc')
      | text(0.55, 0.3,'\alpha\beta0','texmode','on')
  dq0 : Outport  VectorParamsAs1DForOutWhenUnconnected=off
  wires:
  wt/1 -> Alpha-Beta-Zero to dq0/2
  abc/1 -> abc to Alpha-Beta-Zero/1(abc)
  Alpha-Beta-Zero to dq0/1 -> dq0/1
  abc to Alpha-Beta-Zero/1(al_be_0) -> Alpha-Beta-Zero to dq0/1

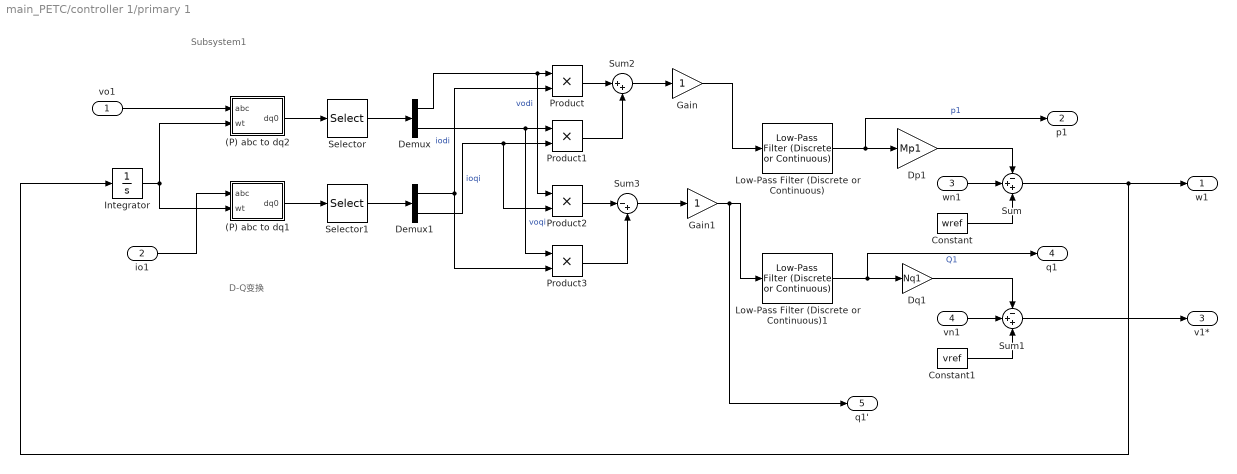
== system main_PETC/controller 1/primary 1 ==
  note: Subsystem1
  note: D-Q变换
  vo1 : Inport
  io1 : Inport  Port=2
  wn1 : Inport  Port=3
  vn1 : Inport  Port=4
  (P) abc to dq1 : Subsystem  AncestorBlock=powerlib_meascontrol/Transformations/abc to dq0  DialogController=POWERSYS.PowerSysDialog  LoadFcn=sps_rtmsupport('LoadFcn', gcbh);  StartFcn=sps_rtmsupport('StartFcn', gcbh);  StopFcn=sps_rtmsupport('StopFcn', gcbh);  mask(abc to dq0 Transformation){Alignment=90 degrees behind phase A axis}
      mask prompts: Alignment "Rotating frame alignment at wt=0:"
      mask help:
      | Perform a Park transformation from a three-phase (abc) signal to a dq0 rotating reference frame. Angular position of the rotating frame is given by input wt (rad).
      |
      | When the rotating frame alignment at wt=0 is 90 degrees behind phase A axis, a positive-sequence signal with Mag=1 & Phase=0 degrees yields the following dq values: d=1, q=0.
      mask init:
      | str=cat(2,gcb,'/Alpha-Beta-Zero to dq0');
      | if Alignment==1
      |     set_param(str,'Alignment','Aligned with phase A axis');
      | else
      |     set_param(str,'Alignment','90 degrees behind phase A axis');
      | end
      settings: CopyFcn=sps_rtmsupport('CopyFcn', gcbh);  DeleteFcn=sps_rtmsupport('DeleteFcn', gcbh);  UndoDeleteFcn=sps_rtmsupport('UndoDeleteFcn', gcbh);  ModelCloseFcn=sps_rtmsupport('ModelCloseFcn', gcbh);  PreSaveFcn=sps_rtmsupport('PreSaveFcn', gcbh);  PostSaveFcn=sps_rtmsupport('PostSaveFcn', gcbh);  NameChangeFcn=sps_rtmsupport('NameChangeFcn', gcbh);  PreCopyFcn=sps_rtmsupport('PreCopyFcn', gcbh);  OpenFcn=sps_rtmsupport('OpenFcn', gcbh, [1]);  CloseFcn=sps_rtmsupport('CloseFcn', gcbh);  PreDeleteFcn=sps_rtmsupport('PreDeleteFcn', gcbh);
      mask Help: helpview(psbhelp);
      mask TypeOptions Alignment: Aligned with phase A axis | 90 degrees behind phase A axis
      mask Display:
      | plot([0 1], [0,1])
      | port_label('input', 1, 'abc')
      | port_label('input', 2, 'wt')
      | port_label('output', 1, 'dq0')
  (P) abc to dq2 : Subsystem  AncestorBlock=powerlib_meascontrol/Transformations/abc to dq0  DialogController=POWERSYS.PowerSysDialog  LoadFcn=sps_rtmsupport('LoadFcn', gcbh);  StartFcn=sps_rtmsupport('StartFcn', gcbh);  StopFcn=sps_rtmsupport('StopFcn', gcbh);  mask(abc to dq0 Transformation){Alignment=90 degrees behind phase A axis}
      mask prompts: Alignment "Rotating frame alignment at wt=0:"
      mask help:
      | Perform a Park transformation from a three-phase (abc) signal to a dq0 rotating reference frame. Angular position of the rotating frame is given by input wt (rad).
      |
      | When the rotating frame alignment at wt=0 is 90 degrees behind phase A axis, a positive-sequence signal with Mag=1 & Phase=0 degrees yields the following dq values: d=1, q=0.
      mask init:
      | str=cat(2,gcb,'/Alpha-Beta-Zero to dq0');
      | if Alignment==1
      |     set_param(str,'Alignment','Aligned with phase A axis');
      | else
      |     set_param(str,'Alignment','90 degrees behind phase A axis');
      | end
      settings: CopyFcn=sps_rtmsupport('CopyFcn', gcbh);  DeleteFcn=sps_rtmsupport('DeleteFcn', gcbh);  UndoDeleteFcn=sps_rtmsupport('UndoDeleteFcn', gcbh);  ModelCloseFcn=sps_rtmsupport('ModelCloseFcn', gcbh);  PreSaveFcn=sps_rtmsupport('PreSaveFcn', gcbh);  PostSaveFcn=sps_rtmsupport('PostSaveFcn', gcbh);  NameChangeFcn=sps_rtmsupport('NameChangeFcn', gcbh);  PreCopyFcn=sps_rtmsupport('PreCopyFcn', gcbh);  OpenFcn=sps_rtmsupport('OpenFcn', gcbh, [1]);  CloseFcn=sps_rtmsupport('CloseFcn', gcbh);  PreDeleteFcn=sps_rtmsupport('PreDeleteFcn', gcbh);
      mask Help: helpview(psbhelp);
      mask TypeOptions Alignment: Aligned with phase A axis | 90 degrees behind phase A axis
      mask Display:
      | plot([0 1], [0,1])
      | port_label('input', 1, 'abc')
      | port_label('input', 2, 'wt')
      | port_label('output', 1, 'dq0')
  Constant : Constant  Value=wref
  Constant1 : Constant  Value=vref
  Demux : Demux  Outputs=2
  Demux1 : Demux  Outputs=2
  Dp1 : Gain  Gain=Mp1
  Dq1 : Gain  Gain=Nq1
  Gain : Gain
  Gain1 : Gain
  Integrator : Integrator
  Low-Pass Filter (Discrete or Continuous) : eeGeneralControl/Low-Pass Filter (Discrete or Continuous)  K=1  T=1/wc  B=inf  A=-inf  init_option=Inherited from block input  x0=0  Ts=-1
  Low-Pass Filter (Discrete or Continuous)1 : eeGeneralControl/Low-Pass Filter (Discrete or Continuous)  K=1  T=1/wc  B=inf  A=-inf  init_option=Inherited from block input  x0=0  Ts=-1
  Product{,1..3} (4 alike) : Product
  Selector : Selector  InputPortWidth=3  IndexOptions=Index vector (dialog)  Indices=[1 2]  OutputSizes=1
  Selector1 : Selector  InputPortWidth=3  IndexOptions=Index vector (dialog)  Indices=[1 2]  OutputSizes=1
  Sum : Sum  Inputs=-++
  Sum1 : Sum  Inputs=-++
  Sum2 : Sum  Inputs=|++
  Sum3 : Sum  Inputs=|-+
  w1 : Outport
  p1 : Outport  Port=2
  v1* : Outport  Port=3
  q1 : Outport  Port=4
  q1' : Outport  Port=5
  wires:
  Low-Pass Filter (Discrete or Continuous)/1 -> Dp1/1, p1/1  "p1"
  Dp1/1 -> Sum/1
  wn1/1 -> Sum/2
  Sum/1 -> Integrator/1, w1/1
  Dq1/1 -> Sum1/1
  Low-Pass Filter (Discrete or Continuous)1/1 -> Dq1/1, q1/1  "Q1"
  Sum1/1 -> v1*/1
  vn1/1 -> Sum1/2
  Constant1/1 -> Sum1/3
  Constant/1 -> Sum/3
  Gain1/1 -> q1'/1, Low-Pass Filter (Discrete or Continuous)1/1
  Gain/1 -> Low-Pass Filter (Discrete or Continuous)/1
  Sum3/1 -> Gain1/1
  Sum2/1 -> Gain/1
  vo1/1 -> (P) abc to dq2/1(abc)
  io1/1 -> (P) abc to dq1/1(abc)
  Product/1 -> Sum2/1
  Product1/1 -> Sum2/2
  Demux1/2 -> Product1/2, Product2/2  "ioqi"
  Product2/1 -> Sum3/1
  Product3/1 -> Sum3/2
  (P) abc to dq1/1(dq0) -> Selector1/1
  Demux1/1 -> Product3/2, Product/2  "iodi"
  (P) abc to dq2/1(dq0) -> Selector/1
  Demux/1 -> Product2/1, Product/1  "vodi"
  Integrator/1 -> (P) abc to dq1/2(wt), (P) abc to dq2/2(wt)
  Selector1/1 -> Demux1/1
  Demux/2 -> Product1/1, Product3/1  "voqi"
  Selector/1 -> Demux/1

== system main_PETC/controller 1/v_secondary 1 ==
  q1' : Inport
  Constant : Constant  Value=wc
  Gain1 : Gain  Gain=wc
  Gain11 : Gain  Gain=Nq1
  Gain5 : Gain  Gain=cv
  Integrator : Integrator  ExternalReset=rising
  Product : Product
  Step : Step  Time=t2  SampleTime=0
  Sum : Sum  Inputs=|+-
  Sum5 : Sum  Inputs=|++
  vn1 : Outport
  wires:
  [zv1] -> Gain5/1
  q1'/1 -> Product/1
  Constant/1 -> Product/2
  Product/1 -> Sum/1
  Gain1/1 -> Sum/2
  [q1] -> Gain1/1
  Sum/1 -> Gain11/1
  Gain5/1 -> Sum5/1
  Gain11/1 -> Sum5/2
  Sum5/1 -> Integrator/1
  Step/1 -> Integrator/2
  Integrator/1 -> vn1/1

== system main_PETC/controller 1/w_secondary 1 ==
  Gain : Gain  Gain=cw
  Gain15 : Gain  Gain=cp
  Integrator : Integrator  ExternalReset=rising
  Step : Step  Time=t2  SampleTime=0
  Sum6 : Sum  Inputs=++|
  wn1 : Outport
  wires:
  Sum6/1 -> Integrator/1
  Gain15/1 -> Sum6/2
  Integrator/1 -> wn1/1
  [zw1] -> Gain/1
  Gain/1 -> Sum6/1
  [zp1] -> Gain15/1
  Step/1 -> Integrator/2

== system main_PETC/controller 2/(P) abc to dq2 ==
  abc : Inport  PortDimensions=3
  wt : Inport  Port=2  PortDimensions=1
  Alpha-Beta-Zero to dq0 : spsAlphaBetaZerotodq0Lib/Alpha-Beta-Zero to dq0  Alignment=90 degrees behind phase A axis
      settings: SourceProductBaseCode=PS
  abc to Alpha-Beta-Zero : Subsystem  AncestorBlock=powerlib_meascontrol/Transformations/abc to Alpha-Beta-Zero  DialogController=POWERSYS.PowerSysDialog  LoadFcn=sps_rtmsupport('LoadFcn', gcbh);  StartFcn=sps_rtmsupport('StartFcn', gcbh);  StopFcn=sps_rtmsupport('StopFcn', gcbh);  mask(abc to Alpha-Beta-Zero Transformation){}
      mask help: Perform a Clarke transformation from a three-phase (abc) signal to a alpha-beta-zero stationary reference frame.
      settings: CopyFcn=sps_rtmsupport('CopyFcn', gcbh);  DeleteFcn=sps_rtmsupport('DeleteFcn', gcbh);  UndoDeleteFcn=sps_rtmsupport('UndoDeleteFcn', gcbh);  ModelCloseFcn=sps_rtmsupport('ModelCloseFcn', gcbh);  PreSaveFcn=sps_rtmsupport('PreSaveFcn', gcbh);  PostSaveFcn=sps_rtmsupport('PostSaveFcn', gcbh);  NameChangeFcn=sps_rtmsupport('NameChangeFcn', gcbh);  PreCopyFcn=sps_rtmsupport('PreCopyFcn', gcbh);  OpenFcn=sps_rtmsupport('OpenFcn', gcbh, []);  CloseFcn=sps_rtmsupport('CloseFcn', gcbh);  PreDeleteFcn=sps_rtmsupport('PreDeleteFcn', gcbh);
      mask Help: helpview(psbhelp);
      mask Display:
      | plot([0 1], [0,1])
      | text(0.15,0.7,'abc')
      | text(0.55, 0.3,'\alpha\beta0','texmode','on')
  dq0 : Outport  VectorParamsAs1DForOutWhenUnconnected=off
  wires:
  wt/1 -> Alpha-Beta-Zero to dq0/2
  abc/1 -> abc to Alpha-Beta-Zero/1(abc)
  Alpha-Beta-Zero to dq0/1 -> dq0/1
  abc to Alpha-Beta-Zero/1(al_be_0) -> Alpha-Beta-Zero to dq0/1

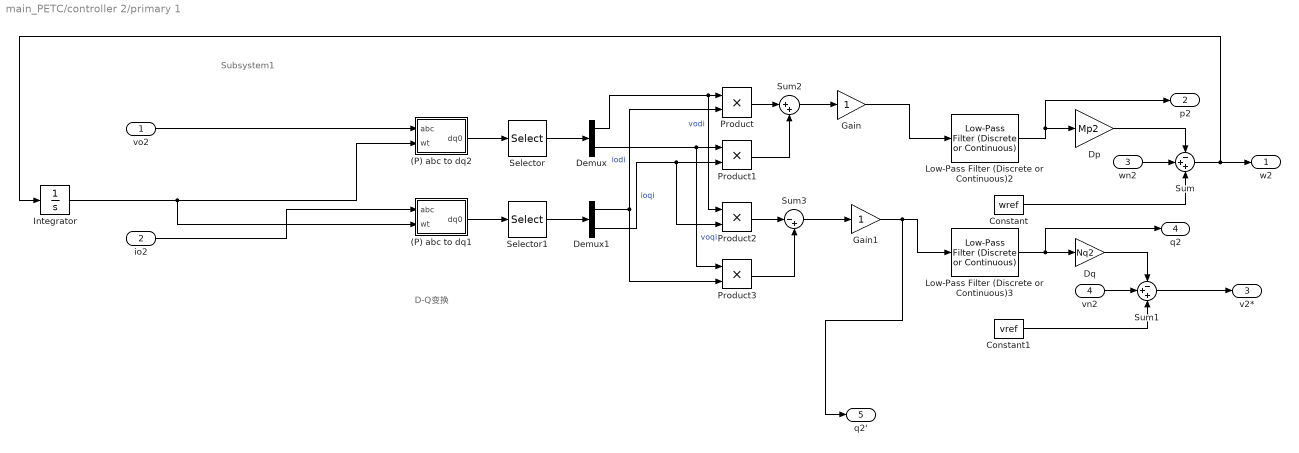
== system main_PETC/controller 2/primary 1 ==
  note: Subsystem1
  note: D-Q变换
  vo2 : Inport
  io2 : Inport  Port=2
  wn2 : Inport  Port=3
  vn2 : Inport  Port=4
  (P) abc to dq1 : Subsystem  AncestorBlock=powerlib_meascontrol/Transformations/abc to dq0  DialogController=POWERSYS.PowerSysDialog  LoadFcn=sps_rtmsupport('LoadFcn', gcbh);  StartFcn=sps_rtmsupport('StartFcn', gcbh);  StopFcn=sps_rtmsupport('StopFcn', gcbh);  mask(abc to dq0 Transformation){Alignment=90 degrees behind phase A axis}
      mask prompts: Alignment "Rotating frame alignment at wt=0:"
      mask help:
      | Perform a Park transformation from a three-phase (abc) signal to a dq0 rotating reference frame. Angular position of the rotating frame is given by input wt (rad).
      |
      | When the rotating frame alignment at wt=0 is 90 degrees behind phase A axis, a positive-sequence signal with Mag=1 & Phase=0 degrees yields the following dq values: d=1, q=0.
      mask init:
      | str=cat(2,gcb,'/Alpha-Beta-Zero to dq0');
      | if Alignment==1
      |     set_param(str,'Alignment','Aligned with phase A axis');
      | else
      |     set_param(str,'Alignment','90 degrees behind phase A axis');
      | end
      settings: CopyFcn=sps_rtmsupport('CopyFcn', gcbh);  DeleteFcn=sps_rtmsupport('DeleteFcn', gcbh);  UndoDeleteFcn=sps_rtmsupport('UndoDeleteFcn', gcbh);  ModelCloseFcn=sps_rtmsupport('ModelCloseFcn', gcbh);  PreSaveFcn=sps_rtmsupport('PreSaveFcn', gcbh);  PostSaveFcn=sps_rtmsupport('PostSaveFcn', gcbh);  NameChangeFcn=sps_rtmsupport('NameChangeFcn', gcbh);  PreCopyFcn=sps_rtmsupport('PreCopyFcn', gcbh);  OpenFcn=sps_rtmsupport('OpenFcn', gcbh, [1]);  CloseFcn=sps_rtmsupport('CloseFcn', gcbh);  PreDeleteFcn=sps_rtmsupport('PreDeleteFcn', gcbh);
      mask Help: helpview(psbhelp);
      mask TypeOptions Alignment: Aligned with phase A axis | 90 degrees behind phase A axis
      mask Display:
      | plot([0 1], [0,1])
      | port_label('input', 1, 'abc')
      | port_label('input', 2, 'wt')
      | port_label('output', 1, 'dq0')
  (P) abc to dq2 : Subsystem  AncestorBlock=powerlib_meascontrol/Transformations/abc to dq0  DialogController=POWERSYS.PowerSysDialog  LoadFcn=sps_rtmsupport('LoadFcn', gcbh);  StartFcn=sps_rtmsupport('StartFcn', gcbh);  StopFcn=sps_rtmsupport('StopFcn', gcbh);  mask(abc to dq0 Transformation){Alignment=90 degrees behind phase A axis}
      mask prompts: Alignment "Rotating frame alignment at wt=0:"
      mask help:
      | Perform a Park transformation from a three-phase (abc) signal to a dq0 rotating reference frame. Angular position of the rotating frame is given by input wt (rad).
      |
      | When the rotating frame alignment at wt=0 is 90 degrees behind phase A axis, a positive-sequence signal with Mag=1 & Phase=0 degrees yields the following dq values: d=1, q=0.
      mask init:
      | str=cat(2,gcb,'/Alpha-Beta-Zero to dq0');
      | if Alignment==1
      |     set_param(str,'Alignment','Aligned with phase A axis');
      | else
      |     set_param(str,'Alignment','90 degrees behind phase A axis');
      | end
      settings: CopyFcn=sps_rtmsupport('CopyFcn', gcbh);  DeleteFcn=sps_rtmsupport('DeleteFcn', gcbh);  UndoDeleteFcn=sps_rtmsupport('UndoDeleteFcn', gcbh);  ModelCloseFcn=sps_rtmsupport('ModelCloseFcn', gcbh);  PreSaveFcn=sps_rtmsupport('PreSaveFcn', gcbh);  PostSaveFcn=sps_rtmsupport('PostSaveFcn', gcbh);  NameChangeFcn=sps_rtmsupport('NameChangeFcn', gcbh);  PreCopyFcn=sps_rtmsupport('PreCopyFcn', gcbh);  OpenFcn=sps_rtmsupport('OpenFcn', gcbh, [1]);  CloseFcn=sps_rtmsupport('CloseFcn', gcbh);  PreDeleteFcn=sps_rtmsupport('PreDeleteFcn', gcbh);
      mask Help: helpview(psbhelp);
      mask TypeOptions Alignment: Aligned with phase A axis | 90 degrees behind phase A axis
      mask Display:
      | plot([0 1], [0,1])
      | port_label('input', 1, 'abc')
      | port_label('input', 2, 'wt')
      | port_label('output', 1, 'dq0')
  Constant : Constant  Value=wref
  Constant1 : Constant  Value=vref
  Demux : Demux  Outputs=2
  Demux1 : Demux  Outputs=2
  Dp : Gain  Gain=Mp2
  Dq : Gain  Gain=Nq2
  Gain : Gain
  Gain1 : Gain
  Integrator : Integrator
  Low-Pass Filter (Discrete or Continuous)2 : eeGeneralControl/Low-Pass Filter (Discrete or Continuous)  K=1  T=1/wc  B=inf  A=-inf  init_option=Inherited from block input  x0=0  Ts=-1
  Low-Pass Filter (Discrete or Continuous)3 : eeGeneralControl/Low-Pass Filter (Discrete or Continuous)  K=1  T=1/wc  B=inf  A=-inf  init_option=Inherited from block input  x0=0  Ts=-1
  Product{,1..3} (4 alike) : Product
  Selector : Selector  InputPortWidth=3  IndexOptions=Index vector (dialog)  Indices=[1 2]  OutputSizes=1
  Selector1 : Selector  InputPortWidth=3  IndexOptions=Index vector (dialog)  Indices=[1 2]  OutputSizes=1
  Sum : Sum  Inputs=-++
  Sum1 : Sum  Inputs=-++
  Sum2 : Sum  Inputs=|++
  Sum3 : Sum  Inputs=|-+
  w2 : Outport
  p2 : Outport  Port=2
  v2* : Outport  Port=3
  q2 : Outport  Port=4
  q2' : Outport  Port=5
  wires:
  vn2/1 -> Sum1/2
  Constant/1 -> Sum/3
  Sum1/1 -> v2*/1
  Constant1/1 -> Sum1/3
  Low-Pass Filter (Discrete or Continuous)3/1 -> Dq/1, q2/1
  Sum/1 -> w2/1, Integrator/1
  Dq/1 -> Sum1/1
  wn2/1 -> Sum/2
  Dp/1 -> Sum/1
  Low-Pass Filter (Discrete or Continuous)2/1 -> Dp/1, p2/1
  Gain1/1 -> q2'/1, Low-Pass Filter (Discrete or Continuous)3/1
  Gain/1 -> Low-Pass Filter (Discrete or Continuous)2/1
  Sum3/1 -> Gain1/1
  Sum2/1 -> Gain/1
  vo2/1 -> (P) abc to dq2/1(abc)
  io2/1 -> (P) abc to dq1/1(abc)
  Product/1 -> Sum2/1
  Product1/1 -> Sum2/2
  Demux1/2 -> Product1/2, Product2/2  "ioqi"
  Product2/1 -> Sum3/1
  Product3/1 -> Sum3/2
  (P) abc to dq1/1(dq0) -> Selector1/1
  Demux1/1 -> Product3/2, Product/2  "iodi"
  (P) abc to dq2/1(dq0) -> Selector/1
  Demux/1 -> Product2/1, Product/1  "vodi"
  Integrator/1 -> (P) abc to dq1/2(wt), (P) abc to dq2/2(wt)
  Selector1/1 -> Demux1/1
  Demux/2 -> Product1/1, Product3/1  "voqi"
  Selector/1 -> Demux/1
